simulink model "Maruti_Swift_Desire_Model_Rhyni"  (R2023a)
settings: Solver=ode45  StartTime=0.0  StopTime=10  RelTol=1e-3  EnableMultiTasking=on
undefined symbols (not defined in the file): magnitude
libraries: simulink x1
settings Model: Creator=INTEL  LastModifiedBy=vashe
settings SolverCC: AlgebraicLoopSolver=TrustRegion
settings DataIOCC: LimitDataPoints=on  SaveFormat=Array  ReturnWorkspaceOutputs=off  Refine=50
settings OptimizationCC: LifeSpan=inf
settings DebuggingCC: SolverPrmCheckMsg=warning  UnconnectedInputMsg=warning  UnconnectedOutputMsg=warning  UnconnectedLineMsg=warning  SFUnexpectedBacktrackingDiag=warning  SFNoUnconditionalDefaultTransitionDiag=warning  SFExecutionAtInitializationDiag=none  ArithmeticOperatorsInVariantConditions=warning
settings HardwareCC: ProdBitPerPointer=32  ProdBitPerSizeT=32  ProdBitPerPtrDiffT=32  ProdLargestAtomicFloat=None  ProdIntDivRoundTo=Undefined  ProdEndianess=Unspecified  ProdWordSize=32  ProdHWDeviceType=32-bit Generic
settings ModelReferenceCC: PropagateSignalLabelsOutOfModel=off
settings SFSimCC: SimUseLocalCustomCode=off  CustomCodeUndefinedFunction=UseInterfaceOnly
settings RTWCC: RTWUseLocalCustomCode=off
settings CodeAppCC: StateflowObjectComments=on
settings GRTTargetCC: TargetLangStandard=C89/C90 (ANSI)
settings ConfigComp: CovMetricSettings=dw  CovSaveCumulativeToWorkspaceVar=on  CovSaveSingleToWorkspaceVar=on  CovExternalEMLEnable=off  CovSFcnEnable=off

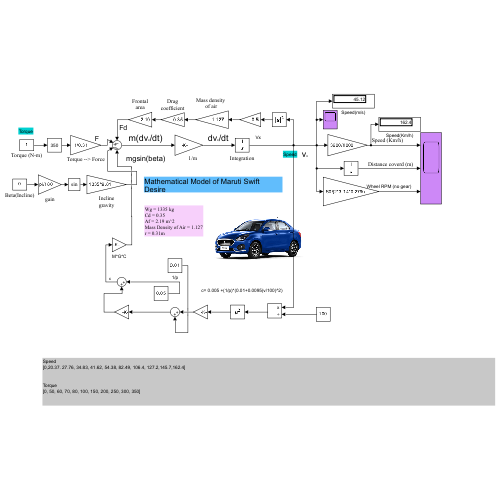
[thumbnail: Simulink's stored preview of the top-level diagram]
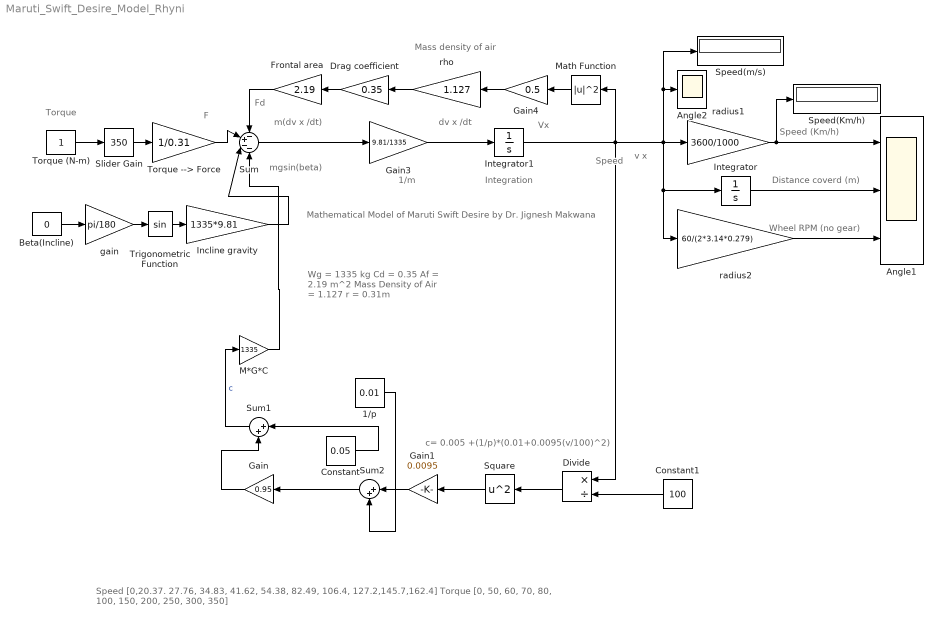
== system Maruti_Swift_Desire_Model_Rhyni ==
  note: c= 0.005 +(1/p)*(0.01+0.0095(v/100)^2)
  note: Vx
  note: Mathematical Model of Maruti Swift Desire
      | by Dr. Jignesh Makwana
  note: v x
  note: Speed
  note: Mass density
      | of air
  note: 1/m
  note: Integration
  note: F
  note: Fd
  note: mgsin(beta)
  note: Distance coverd (m)
  note: Speed (Km/h)
  note: Wheel RPM (no gear)
  note: Torque
  note: dv x /dt
  note: m(dv x /dt)
  note: Wg = 1335 kg
      | Cd = 0.35
      | Af = 2.19 m^2
      | Mass Density of Air = 1.127
      | r = 0.31m
  note: Speed
      | [0,20.37. 27.76, 34.83, 41.62, 54.38, 82.49, 106.4, 127.2,145.7,162.4]
      |
      |
      | Torque
      | [0, 50, 60, 70, 80, 100, 150, 200, 250, 300, 350]
  1/p : Constant  Value=0.01
  Angle1 : Scope  NumInputPorts=3
  Angle2 : Scope
  Beta(Incline) : Constant  Value=0
  Constant : Constant  Value=0.05
  Constant1 : Constant  Value=100
  Divide : Product  Inputs=*/
  Drag coefficient : Gain  Gain=0.35
  Frontal area : Gain  Gain=2.19
  Gain : Gain  Gain=0.95
  Gain1 : Gain  Gain=0.0095
  Gain3 : Gain  Gain=9.81/1335
  Gain4 : Gain  Gain=0.5
  Incline gravity : Gain  Gain=1335*9.81
  Integrator : Integrator
  Integrator1 : Integrator
  M*G*C : Gain  Gain=1335
  Math Function : Math  Operator=magnitude^2  SignedPower=on
  Slider Gain : simulink/Math Operations/Slider Gain  gain=350  low=0  high=400
  Speed(Km/h) : Display
  Speed(m/s) : Display
  Square : Math  Operator=square
  Sum : Sum  Inputs=-+--
  Sum1 : Sum  Inputs=|++
  Sum2 : Sum  Inputs=|++
  Torque (N-m) : Constant
  Torque --> Force : Gain  Gain=1/0.31
  Trigonometric Function : Trigonometry
  gain : Gain  Gain=pi/180
  radius1 : Gain  Gain=3600/1000
  radius2 : Gain  Gain=60/(2*3.14*0.279)
  rho : Gain  Gain=1.127
  wires:
  Math Function/1 -> Gain4/1
  Frontal area/1 -> Sum/1
  Drag coefficient/1 -> Frontal area/1
  rho/1 -> Drag coefficient/1
  Gain4/1 -> rho/1
  Incline gravity/1 -> Sum/3
  Trigonometric Function/1 -> Incline gravity/1
  Gain3/1 -> Integrator1/1
  Sum/1 -> Gain3/1
  radius1/1 -> Speed(Km/h)/1, Angle1/1
  Integrator/1 -> Angle1/2
  radius2/1 -> Angle1/3
  Integrator1/1 -> Math Function/1, Divide/1, Speed(m/s)/1, Angle2/1, radius1/1, Integrator/1, radius2/1
  Torque --> Force/1 -> Sum/2
  Beta(Incline)/1 -> gain/1
  gain/1 -> Trigonometric Function/1
  Torque (N-m)/1 -> Slider Gain/1
  Slider Gain/1 -> Torque --> Force/1
  Constant/1 -> Sum1/1
  Gain/1 -> Sum1/2
  Divide/1 -> Square/1
  Square/1 -> Gain1/1
  Constant1/1 -> Divide/2
  Gain1/1 -> Sum2/1
  1/p/1 -> Sum2/2
  Sum2/1 -> Gain/1
  Sum1/1 -> M*G*C/1  "c"
  M*G*C/1 -> Sum/4
